simulink model "Phase1_simulink"  (R2021b)
settings: Solver=VariableStepAuto  StartTime=0.0  StopTime=1  RelTol=1e-3
values from neighbouring files (symbols this model uses):
  A_eq = double(A_eq)    [source_export.m]
  B_eq = double(B_eq)    [source_export.m]
  C = [1 0 0 0 0 0 0 0 0 0 0 0 ... (first row only)    [source_export.m]
  C_simulink = eye(12)    [source_export.m]
  Condition_0 = transpose([0 0 0 0 0 0 0 0 0 0 0 0])    [source_export.m]
  Condition_1 = transpose([0.2 0.2 0.2 0.2 0.2 0.2 0.2 0.2 0.2 0.2 0.2 0.2])    [source_export.m]
  D = zeros(4,4)    [source_export.m]
  D_Simulink = zeros(12,4)    [source_export.m]
  g = 9.81    [source_export.m]
  Ixx = 0.0035    [source_export.m]
  Iyy = 0.0035    [source_export.m]
  Izz = 0.005    [source_export.m]
  m = 1    [source_export.m]
settings Model: Creator=ali14  LastModifiedBy=Arian
settings DebuggingCC: UnconnectedInputMsg=none  UnconnectedOutputMsg=none  UnconnectedLineMsg=none
settings ModelReferenceCC: EnableRefExpFcnMdlSchedulingChecks=off
settings RTWCC: DLArmComputeVersion=20.02.1

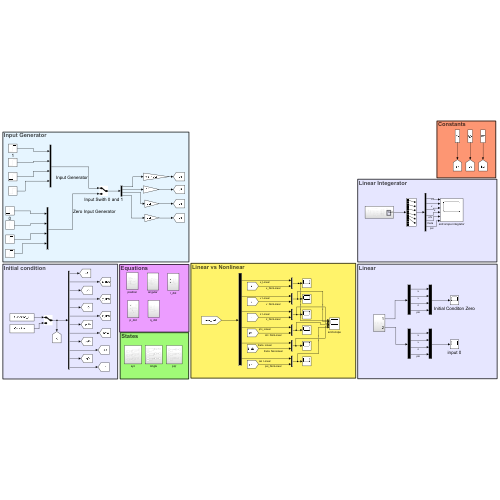
[thumbnail: Simulink's stored preview of the top-level diagram]
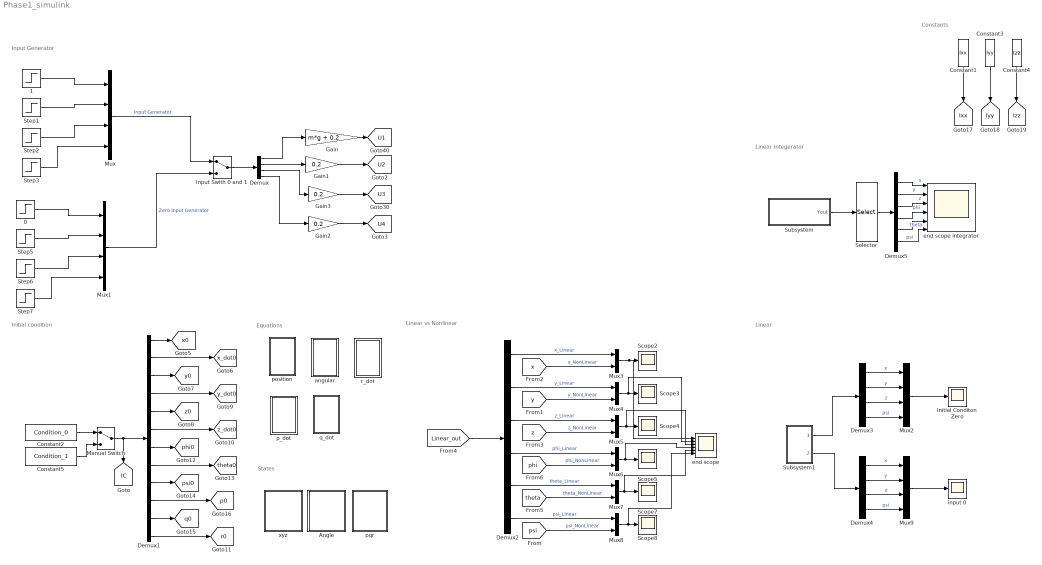
== system Phase1_simulink ==
  note: Linear Integerator
  note: Input Generator
  note: Linear
  note: Linear vs Nonlinear
  note: Constants
  note: Initial condition
  note: States
  note: Equations
  0 : Step  Time=0  After=0  SampleTime=0
  1 : Step  Time=0  SampleTime=0
  Angle : Subsystem
  Constant1 : Constant  Value=Ixx
  Constant2 : Constant  Value=Condition_0
  Constant3 : Constant  Value=Iyy
  Constant4 : Constant  Value=Izz
  Constant5 : Constant  Value=Condition_1  VectorParams1D=off
  Demux : Demux
  Demux1 : Demux  Outputs=12
  Demux2 : Demux  Outputs=6
  Demux3 : Demux
  Demux4 : Demux
  Demux5 : Demux  Outputs=6
  Gain : Gain  Gain=m*g + 0.2
  Gain1 : Gain  Gain=0.2
  Gain2 : Gain  Gain=0.2
  Gain3 : Gain  Gain=0.2
  Initial Conditon Zero : Scope
  Input Swith 0 and 1 : ManualSwitch
  Manual Switch : ManualSwitch
  Mux{,1..2,9} (4 alike) : Mux
  Mux{3..8} (6 alike) : Mux  Inputs=2
  Scope{2..5,7..8} (6 alike) : Scope
  Selector : Selector  InputPortWidth=12  IndexOptions=Index vector (dialog)  Indices=[1 3 5 7 8 9]  OutputSizes=1
  Step1 : Step  Time=0  SampleTime=0
  Step2 : Step  Time=0  SampleTime=0
  Step3 : Step  Time=0  SampleTime=0
  Step5 : Step  Time=0  After=0  SampleTime=0
  Step6 : Step  Time=0  After=0  SampleTime=0
  Step7 : Step  Time=0  After=0  SampleTime=0
  Subsystem : Subsystem
  Subsystem1 : Subsystem
  angular : Subsystem
  end scope : Scope  NumInputPorts=6
  end scope integrator : Scope  NumInputPorts=6
  input 0 : Scope
  p_dot : Subsystem
  position : Subsystem
  pqr : Subsystem
  q_dot : Subsystem
  r_dot : Subsystem
  xyz : Subsystem
  tag scope: IC=global, Ixx=global, Iyy=global, Izz=global, U1=global, U2=global, U3=global, U4=global, p0=global, phi0=global, psi0=global, q0=global, r0=global, theta0=global, x0=global, x_dot0=global, y0=global, y_dot0=global, z0=global, z_dot0=global
  wires:
  Demux1/1 -> [x0]
  Demux1/3 -> [y0]
  Demux1/5 -> [z0]
  Demux1/2 -> [x_dot0]
  Demux1/4 -> [y_dot0]
  Demux1/6 -> [z_dot0]
  Demux1/7 -> [phi0]
  Demux1/8 -> [theta0]
  Demux1/9 -> [psi0]
  Demux1/10 -> [p0]
  Demux1/11 -> [q0]
  Demux1/12 -> [r0]
  Constant1/1 -> [Ixx]
  Constant3/1 -> [Iyy]
  Constant4/1 -> [Izz]
  Constant5/1 -> Manual Switch/2
  Manual Switch/1 -> Demux1/1, [IC]
  Constant2/1 -> Manual Switch/1
  1/1 -> Mux/1
  Step1/1 -> Mux/2
  Step2/1 -> Mux/3
  Step3/1 -> Mux/4
  Mux/1 -> Input Swith 0 and 1/1  "Input Generator"
  Input Swith 0 and 1/1 -> Demux/1
  Step7/1 -> Mux1/4
  0/1 -> Mux1/1
  Step5/1 -> Mux1/2
  Step6/1 -> Mux1/3
  Mux1/1 -> Input Swith 0 and 1/2  "Zero Input Generator"
  Demux/1 -> Gain/1
  Demux/2 -> Gain1/1
  Demux/3 -> Gain3/1
  Demux/4 -> Gain2/1
  Gain1/1 -> [U2]
  Gain3/1 -> [U3]
  Gain2/1 -> [U4]
  Gain/1 -> [U1]
  [Linear_out] -> Demux2/1
  Mux3/1 -> end scope/1, Scope2/1
  Demux2/1 -> Mux3/1  "x_Linear"
  [x] -> Mux3/2  "x_NonLinear"
  Demux2/2 -> Mux4/1  "y_Linear"
  Demux2/3 -> Mux5/1  "z_Linear"
  Demux2/4 -> Mux6/1  "phi_Linear"
  Demux2/5 -> Mux7/1  "theta_Linear"
  Demux2/6 -> Mux8/1  "psi_Linear"
  [y] -> Mux4/2  "y_NonLinear"
  [z] -> Mux5/2  "z_NonLinear"
  [phi] -> Mux6/2  "phi_NonLinear"
  [psi] -> Mux8/2  "psi_NonLinear"
  [theta] -> Mux7/2  "theta_NonLinear"
  Mux4/1 -> end scope/2, Scope3/1
  Mux5/1 -> end scope/3, Scope4/1
  Mux6/1 -> end scope/4, Scope5/1
  Mux7/1 -> end scope/5, Scope7/1
  Mux8/1 -> end scope/6, Scope8/1
  Subsystem1/1(Outport) -> Demux3/1
  Demux3/1 -> Mux2/1  "x"
  Demux3/2 -> Mux2/2  "y"
  Demux3/3 -> Mux2/3  "z"
  Demux3/4 -> Mux2/4  "psi"
  Mux2/1 -> Initial Conditon Zero/1
  Demux4/2 -> Mux9/2  "y"
  Demux4/1 -> Mux9/1  "x"
  Demux4/4 -> Mux9/4  "psi"
  Demux4/3 -> Mux9/3  "z"
  Subsystem1/2(Outport1) -> Demux4/1
  Mux9/1 -> input 0/1
  Subsystem/1(Yout) -> Selector/1
  Selector/1 -> Demux5/1
  Demux5/1 -> end scope integrator/1  "x"
  Demux5/2 -> end scope integrator/2  "y"
  Demux5/3 -> end scope integrator/3  "z"
  Demux5/4 -> end scope integrator/4  "phi"
  Demux5/5 -> end scope integrator/5  "theta"
  Demux5/6 -> end scope integrator/6  "psi"

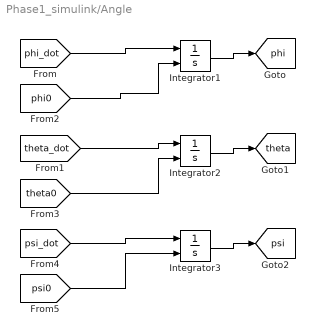
== system Phase1_simulink/Angle ==
  Integrator1 : Integrator  InitialConditionSource=external  WrapState=on
  Integrator2 : Integrator  InitialConditionSource=external  WrapState=on
  Integrator3 : Integrator  InitialConditionSource=external  WrapState=on
  tag scope: phi=global, psi=global, theta=global
  wires:
  Integrator2/1 -> [theta]
  [theta_dot] -> Integrator2/1
  Integrator3/1 -> [psi]
  [theta0] -> Integrator2/2
  [psi_dot] -> Integrator3/1
  [phi0] -> Integrator1/2
  Integrator1/1 -> [phi]
  [psi0] -> Integrator3/2
  [phi_dot] -> Integrator1/1

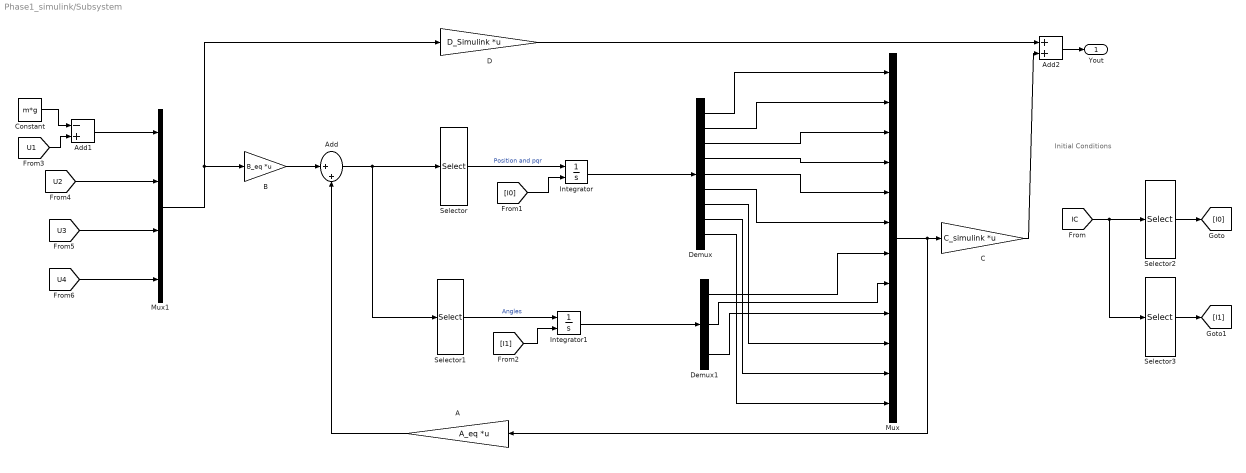
== system Phase1_simulink/Subsystem ==
  note: Initial Conditions
  A : Gain  Gain=A_eq  Multiplication=Matrix(K*u)
  Add : Sum  Inputs=|++
  Add1 : Sum  Inputs=-+
  Add2 : Sum
  B : Gain  Gain=B_eq  Multiplication=Matrix(K*u)
  C : Gain  Gain=C_simulink  Multiplication=Matrix(K*u)
  Constant : Constant  Value=m*g
  D : Gain  Gain=D_Simulink  Multiplication=Matrix(K*u)
  Demux : Demux  Outputs=9
  Demux1 : Demux  Outputs=3
  Integrator : Integrator  InitialConditionSource=external
  Integrator1 : Integrator  InitialConditionSource=external  WrapState=on
  Mux : Mux  Inputs=12
  Mux1 : Mux
  Selector : Selector  InputPortWidth=12  IndexOptions=Index vector (dialog)  Indices=[1 2 3 4 5 6 10 11 12]  OutputSizes=1
  Selector1 : Selector  InputPortWidth=12  IndexOptions=Index vector (dialog)  Indices=[7 8 9]  OutputSizes=1
  Selector2 : Selector  InputPortWidth=12  IndexOptions=Index vector (dialog)  Indices=[1 2 3 4 5 6 10 11 12]  OutputSizes=1
  Selector3 : Selector  InputPortWidth=12  IndexOptions=Index vector (dialog)  Indices=[7 8 9]  OutputSizes=1
  Yout : Outport
  wires:
  B/1 -> Add/1
  A/1 -> Add/2
  Add/1 -> Selector1/1, Selector/1
  Selector/1 -> Integrator/1  "Position and pqr"
  Selector1/1 -> Integrator1/1  "Angles"
  [IC] -> Selector3/1, Selector2/1
  Selector3/1 -> [I1]
  Selector2/1 -> [I0]
  [I1] -> Integrator1/2
  [I0] -> Integrator/2
  Integrator1/1 -> Demux1/1
  Integrator/1 -> Demux/1
  Demux/1 -> Mux/1
  Demux/2 -> Mux/2
  Demux/3 -> Mux/3
  Demux/4 -> Mux/4
  Demux/5 -> Mux/5
  Demux/6 -> Mux/6
  Demux1/1 -> Mux/7
  Demux1/2 -> Mux/8
  Demux1/3 -> Mux/9
  Demux/7 -> Mux/10
  Demux/8 -> Mux/11
  Demux/9 -> Mux/12
  D/1 -> Add2/1
  C/1 -> Add2/2
  Mux1/1 -> D/1, B/1
  [U2] -> Mux1/2
  [U3] -> Mux1/3
  [U4] -> Mux1/4
  Add2/1 -> Yout/1
  Mux/1 -> A/1, C/1
  Constant/1 -> Add1/1
  [U1] -> Add1/2
  Add1/1 -> Mux1/1

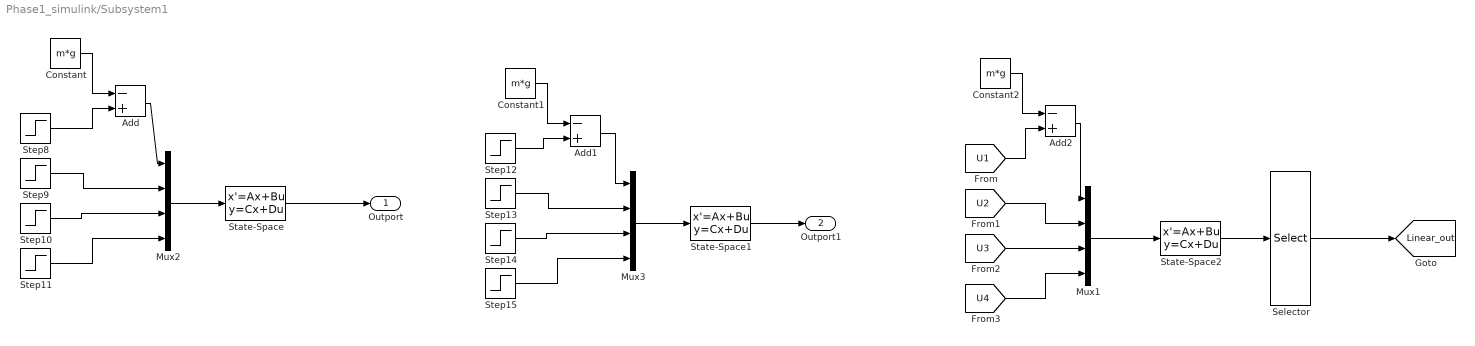
== system Phase1_simulink/Subsystem1 ==
  Add : Sum  Inputs=-+
  Add1 : Sum  Inputs=-+
  Add2 : Sum  Inputs=-+
  Constant : Constant  Value=m*g
  Constant1 : Constant  Value=m*g
  Constant2 : Constant  Value=m*g
  Mux1 : Mux
  Mux2 : Mux
  Mux3 : Mux
  Selector : Selector  InputPortWidth=12  IndexOptions=Index vector (dialog)  Indices=[1 3 5 7 8 9]  OutputSizes=1
  State-Space : StateSpace  A=A_eq  B=B_eq  C=C  D=D  InitialCondition=Condition_0
  State-Space1 : StateSpace  A=A_eq  B=B_eq  C=C  D=D  InitialCondition=Condition_1
  State-Space2 : StateSpace  A=A_eq  B=B_eq  C=C_simulink  D=D_Simulink  InitialCondition=Condition_0  ParameterTunability=Optimized
  Step{8..11} (4 alike) : Step  Time=0  SampleTime=0
  Step{12..15} (4 alike) : Step  Time=0  After=0  SampleTime=0
  Outport : Outport
  Outport1 : Outport  Port=2
  tag scope: Linear_out=global
  wires:
  State-Space1/1 -> Outport1/1
  Step15/1 -> Mux3/4
  Step11/1 -> Mux2/4
  Step9/1 -> Mux2/2
  Mux3/1 -> State-Space1/1
  Step10/1 -> Mux2/3
  State-Space/1 -> Outport/1
  Step13/1 -> Mux3/2
  Mux2/1 -> State-Space/1
  Step14/1 -> Mux3/3
  Mux1/1 -> State-Space2/1
  [U2] -> Mux1/2
  [U3] -> Mux1/3
  [U4] -> Mux1/4
  Constant/1 -> Add/1
  Step8/1 -> Add/2
  Add/1 -> Mux2/1
  Constant1/1 -> Add1/1
  Step12/1 -> Add1/2
  Add1/1 -> Mux3/1
  Constant2/1 -> Add2/1
  [U1] -> Add2/2
  Add2/1 -> Mux1/1
  State-Space2/1 -> Selector/1
  Selector/1 -> [Linear_out]

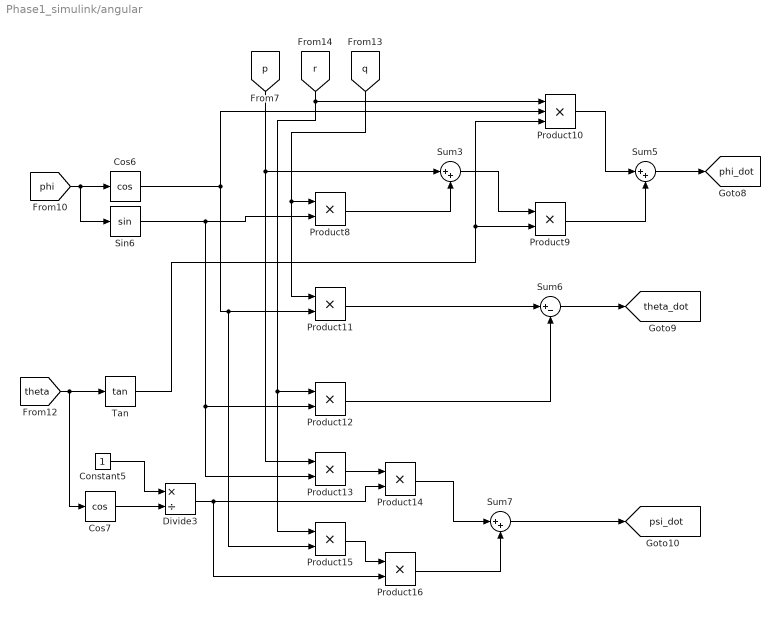
== system Phase1_simulink/angular ==
  Constant5 : Constant
  Cos6 : Trigonometry  Operator=cos
  Cos7 : Trigonometry  Operator=cos
  Divide3 : Product  Inputs=*/
  Product10 : Product  Inputs=3
  Product{8..9,11..16} (8 alike) : Product
  Sin6 : Trigonometry
  Sum3 : Sum  Inputs=|++
  Sum5 : Sum  Inputs=|++
  Sum6 : Sum  Inputs=|+-
  Sum7 : Sum  Inputs=|++
  Tan : Trigonometry  Operator=tan
  tag scope: phi_dot=global, psi_dot=global, theta_dot=global
  wires:
  Product12/1 -> Sum6/2
  [theta] -> Cos7/1, Tan/1
  Product15/1 -> Product16/1
  [p] -> Product13/1, Sum3/1
  [r] -> Product15/1, Product12/1, Product10/1
  [phi] -> Sin6/1, Cos6/1
  Tan/1 -> Product10/3, Product9/2
  Divide3/1 -> Product16/2, Product14/2
  Product14/1 -> Sum7/1
  Sum6/1 -> [theta_dot]
  Sin6/1 -> Product13/2, Product12/2, Product8/2
  Cos6/1 -> Product15/2, Product11/2, Product10/2
  Product9/1 -> Sum5/2
  Product11/1 -> Sum6/1
  Product8/1 -> Sum3/2
  Cos7/1 -> Divide3/2
  [q] -> Product11/1, Product8/1
  Product10/1 -> Sum5/1
  Sum5/1 -> [phi_dot]
  Constant5/1 -> Divide3/1
  Sum7/1 -> [psi_dot]
  Product16/1 -> Sum7/2
  Sum3/1 -> Product9/1
  Product13/1 -> Product14/1

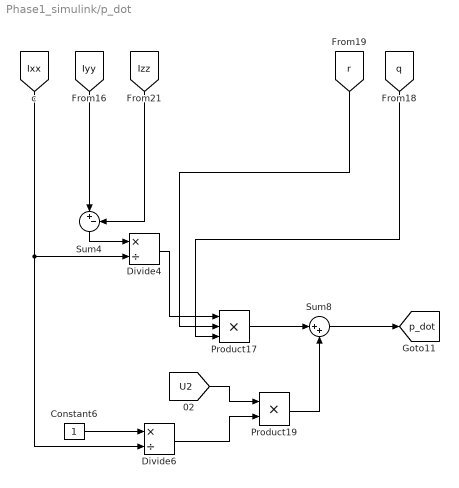
== system Phase1_simulink/p_dot ==
  Constant6 : Constant
  Divide4 : Product  Inputs=*/
  Divide6 : Product  Inputs=*/
  Product17 : Product  Inputs=3
  Product19 : Product
  Sum4 : Sum  Inputs=|+-
  Sum8 : Sum  Inputs=|++
  tag scope: p_dot=global
  wires:
  [Iyy] -> Sum4/1
  [U2] -> Product19/1
  [r] -> Product17/2
  Product19/1 -> Sum8/2
  Divide4/1 -> Product17/1
  [Ixx] -> Divide4/2, Divide6/2
  Product17/1 -> Sum8/1
  [q] -> Product17/3
  Constant6/1 -> Divide6/1
  Divide6/1 -> Product19/2
  Sum4/1 -> Divide4/1
  [Izz] -> Sum4/2
  Sum8/1 -> [p_dot]

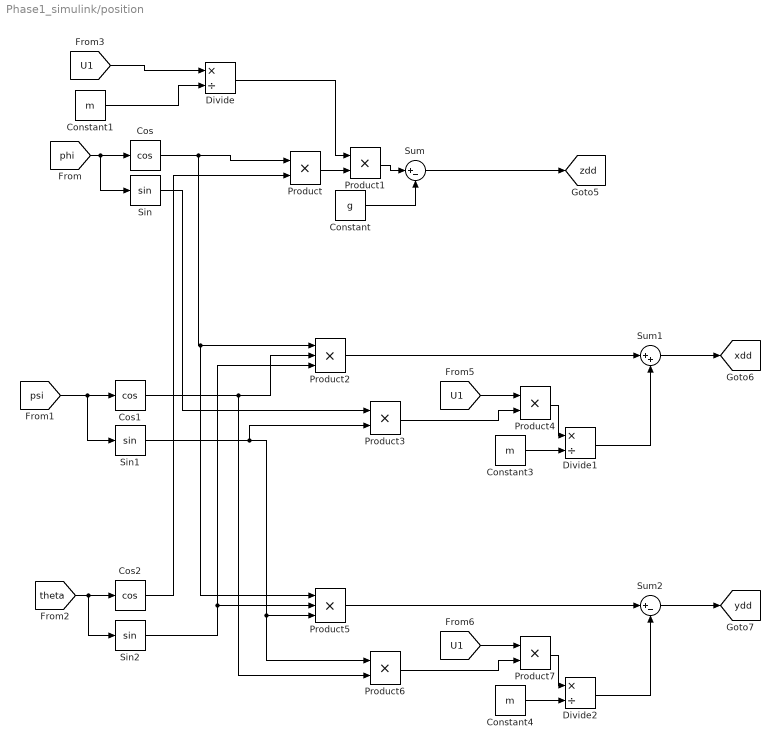
== system Phase1_simulink/position ==
  Constant : Constant  Value=g
  Constant1 : Constant  Value=m
  Constant3 : Constant  Value=m
  Constant4 : Constant  Value=m
  Cos : Trigonometry  Operator=cos
  Cos1 : Trigonometry  Operator=cos
  Cos2 : Trigonometry  Operator=cos
  Divide : Product  Inputs=*/
  Divide1 : Product  Inputs=*/
  Divide2 : Product  Inputs=*/
  Product{,1,3..4,6..7} (6 alike) : Product
  Product2 : Product  Inputs=3
  Product5 : Product  Inputs=3
  Sin : Trigonometry
  Sin1 : Trigonometry
  Sin2 : Trigonometry
  Sum : Sum  Inputs=|+-
  Sum1 : Sum  Inputs=|++
  Sum2 : Sum  Inputs=|+-
  tag scope: xdd=global, ydd=global, zdd=global
  wires:
  Product2/1 -> Sum1/1
  Product7/1 -> Divide2/1
  [psi] -> Sin1/1, Cos1/1
  Product6/1 -> Product7/2
  Divide1/1 -> Sum1/2
  Sin1/1 -> Product3/2, Product6/1, Product5/3
  Cos/1 -> Product5/1, Product2/1, Product/1
  Constant/1 -> Sum/2
  Cos1/1 -> Product6/2, Product2/2
  Cos2/1 -> Product/2
  Sin2/1 -> Product2/3, Product5/2
  Sum2/1 -> [ydd]
  Product5/1 -> Sum2/1
  Sin/1 -> Product3/1
  Divide2/1 -> Sum2/2
  Constant4/1 -> Divide2/2
  [U1] -> Product7/1
  Sum1/1 -> [xdd]
  [phi] -> Sin/1, Cos/1
  [theta] -> Sin2/1, Cos2/1
  Product4/1 -> Divide1/1
  Product3/1 -> Product4/2
  [U1] -> Product4/1
  Constant3/1 -> Divide1/2
  Product1/1 -> Sum/1
  Product/1 -> Product1/2
  Sum/1 -> [zdd]
  Constant1/1 -> Divide/2
  [U1] -> Divide/1
  Divide/1 -> Product1/1

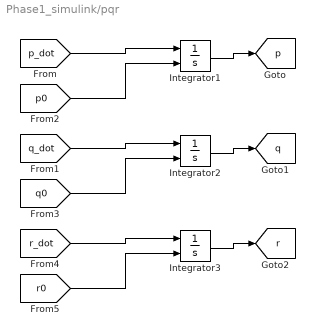
== system Phase1_simulink/pqr ==
  Integrator1 : Integrator  InitialConditionSource=external
  Integrator2 : Integrator  InitialConditionSource=external
  Integrator3 : Integrator  InitialConditionSource=external
  tag scope: p=global, q=global, r=global
  wires:
  [q0] -> Integrator2/2
  [q_dot] -> Integrator2/1
  Integrator2/1 -> [q]
  Integrator1/1 -> [p]
  [p_dot] -> Integrator1/1
  [p0] -> Integrator1/2
  [r_dot] -> Integrator3/1
  [r0] -> Integrator3/2
  Integrator3/1 -> [r]

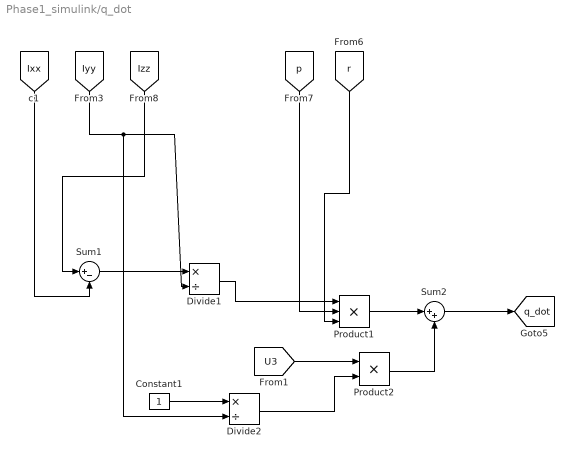
== system Phase1_simulink/q_dot ==
  Constant1 : Constant
  Divide1 : Product  Inputs=*/
  Divide2 : Product  Inputs=*/
  Product1 : Product  Inputs=3
  Product2 : Product
  Sum1 : Sum  Inputs=|+-
  Sum2 : Sum  Inputs=|++
  tag scope: q_dot=global
  wires:
  Sum1/1 -> Divide1/1
  Product1/1 -> Sum2/1
  [Izz] -> Sum1/1
  [Iyy] -> Divide2/2, Divide1/2
  Divide1/1 -> Product1/1
  Product2/1 -> Sum2/2
  Divide2/1 -> Product2/2
  [p] -> Product1/2
  [r] -> Product1/3
  Constant1/1 -> Divide2/1
  [U3] -> Product2/1
  Sum2/1 -> [q_dot]
  [Ixx] -> Sum1/2

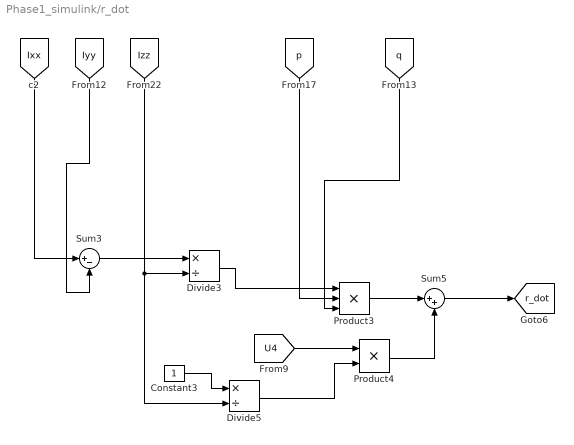
== system Phase1_simulink/r_dot ==
  Constant3 : Constant
  Divide3 : Product  Inputs=*/
  Divide5 : Product  Inputs=*/
  Product3 : Product  Inputs=3
  Product4 : Product
  Sum3 : Sum  Inputs=|+-
  Sum5 : Sum  Inputs=|++
  tag scope: r_dot=global
  wires:
  Constant3/1 -> Divide5/1
  [Ixx] -> Sum3/1
  [q] -> Product3/3
  [Izz] -> Divide5/2, Divide3/2
  Product4/1 -> Sum5/2
  Product3/1 -> Sum5/1
  [U4] -> Product4/1
  [Iyy] -> Sum3/2
  Sum3/1 -> Divide3/1
  Divide3/1 -> Product3/1
  [p] -> Product3/2
  Sum5/1 -> [r_dot]
  Divide5/1 -> Product4/2

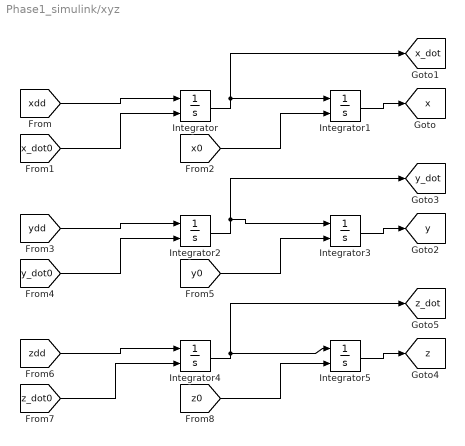
== system Phase1_simulink/xyz ==
  Integrator{,1..5} (6 alike) : Integrator  InitialConditionSource=external
  tag scope: x=global, x_dot=global, y=global, y_dot=global, z=global, z_dot=global
  wires:
  Integrator3/1 -> [y]
  [z0] -> Integrator5/2
  [x0] -> Integrator1/2
  Integrator2/1 -> Integrator3/1, [y_dot]
  [y0] -> Integrator3/2
  Integrator/1 -> Integrator1/1, [x_dot]
  Integrator1/1 -> [x]
  Integrator4/1 -> Integrator5/1, [z_dot]
  Integrator5/1 -> [z]
  [z_dot0] -> Integrator4/2
  [zdd] -> Integrator4/1
  [y_dot0] -> Integrator2/2
  [ydd] -> Integrator2/1
  [x_dot0] -> Integrator/2
  [xdd] -> Integrator/1
